simulink model "Latest_Greatest"  (R2022a)
settings: Solver=ode4  StartTime=0  StopTime=15  FixedStep=DeltaT  RelTol=1e-3  EnableMultiTasking=on
InitFcn:
  | % Dynamics Simulation          DA Cole
  | clear all;close all;clc;warning off all;
  | 
  | open('pitchyaw.mat');
  | 
  | % Simulation run parameters
  | %Rate=34.3;  DeltaT=1/Rate;
  | %Rate=40;  DeltaT=1/Rate;
  | %Rate=100;  DeltaT=1/Rate;
  | %Rate=130; DeltaT=1/Rate;
  | %Rate=90; DeltaT=1/Rate;
  | %Rate=110; DeltaT=1/Rate;
  | %Rate=120; DeltaT=1/Rate;
  | %Rate=115; DeltaT=1/Rate;
  | %Rate=125; DeltaT=1/Rate;
  | Rate=117; DeltaT=1/Rate;
  | 
  | 
  | % Maneuver Parameters
  | roll=10;  pitch=-30; yaw=30;   roll=roll*pi/180; pitch=pitch*pi/180; yaw=yaw*pi/180;
  | SlewTime=5;   SACengage=0;
  | 
  | %Constants0
  | Re=6371.2e3;mu=398601.2e9;          %earth radius and universal gravitation constant
  | 
  | %Spacecraft orbit
  | h=0;                                     %orbit altitude
  | R=Re+h;                             %orbit radius from center of earth
  | we=0.000072921158553;   %earth's angular velocity rad/solar sec(Vallado)
  | wo=sqrt(mu/(Re+h)^3);        %orbit angular velocity
  | incln=36.6001*pi/180;          %Inclination assumed Monterey Latitude
  | epsilon=12*pi/180;  alphao=0;
  | uo=0; nuo=0;                        %Start S/C beneath subsolar point
  | beta=60; gamma=1.5;
  | a=0.545491852; b=0.314939867;  c=0.704226952;   %Assumed spacecraft rectangular size
  | Area=[b*c a*c a*b];                 %projected area~m^2 in body x,y,z directions
  | density=4.39e-14;
  | kpre=-9.9639/24/3600/180*pi*0;      %nodal precession constant assumed zero here
  | wn=kpre*(Re/(Re+h))^3.5*cos(incln); %nodal precession (zero eccentricity)
  | V=wo*(Re+h);
  | rho=asin(Re/(h+Re));                %earth angular radius
  | Cd=2.5;     psun=4.5E-6;            %Drag coefficient and solar pressure constant~N/m^2
  | Kaero=-0.5*Cd*V^2;   Psolar=2*psun;  %constants for aero and solar torque calculation
  | dL=[0.002 0.002 0.008];             %predicted distance between cp and cg
  | Kme=2.3390e-005;
  | 
  | %Spacecraft Magnetic Properties (assumed)
  | mresid=[0 0 0.01];                  %Spacecraft residual magnetic moment
  | M=mresid;                           %Magnetic unit dipole vector
  | K=7.943e15;
  | 
  | % ACTUAL Spacecraft Inertia conditions
  | Ix=90;   Iy=100;   Iz=250 ;
  | Ixy=-10;  Iyz=20;  Ixz=-10;
  | Imo=[Ix -Ixy -Ixz;
  |        -Ixy  Iy  -Iyz;
  |        -Ixz -Iyz  Iz];                  %Moment of inertia matrix
  | Iinv=inv(Imo);                      %Moment of inertia inverse goes in dynamics block
  | 
  | %Spacecraft initial Euler state angles and rates
  | ... (+68 lines)
StopFcn:
  | if flag==0; Hcmg=Hcmg;else;Hcmg=HcmgMP;end;
  | Hxcmg=[];Hycmg=[];Hzcmg=[];CondA=[]; CondA_MP=[];t=[]; SingPt=[];DetA=[];
  | for i=1:max(size(A));  t=[t i*DeltaT];  H=Hcmg(:,:,i); Hx=H(1,:);  Hy=H(2,:);  Hz=H(3,:);
  | detA=det(A(:,1:3,i));Hxcmg=[Hxcmg Hx];  Hycmg=[Hycmg Hy];  Hzcmg=[Hzcmg Hz];
  | CONDA=cond(A(:,:,i));
  | DetA=[DetA detA]; DetA=1./DetA;
  | CondA=[CondA CONDA];end;   %CondA=CondA./max(CondA); DetA=DetA./max(DetA);
  | Hmag=sqrt(Hxcmg.^2+Hycmg.^2+Hzcmg.^2);x=(max(t)-DeltaT);
  | 
  | InvCondA;
  | 
  | if flag==0; MaxInvCond=min(1./CondA(10*Rate+1:end));DELTA=delta;DELTAdot=deltadot;
  | else; MaxInvCond=min(1./CondA_MP(10*Rate+1:end));DELTA=delta_MP;DELTAdot=deltadot_MP;Hcmg=HcmgMP;end;
  | 
  | ERROR=(trajectory*180/pi-Euler);
  | 
  | figure(1); wdotTrajectory=[CMDTrajectory(:,1) CMDTrajectory(:,2) CMDTrajectory(:,3)];  wTrajectory=[CMDTrajectory(:,4) CMDTrajectory(:,5) CMDTrajectory(:,6)]; ThetaTrajectory=180/pi.*[trajectory(:,1) trajectory(:,2) trajectory(:,3)];
  | subplot(3,1,1); plot(t,wdotTrajectory,'linewidth',2); axis tight; grid; ylabel('\omega^d^o^t_C_M_D (deg)','fontsize',16); title('Desired Angle, Rate, Acceleration Trajectories','fontsize',16);   set(gca,'XTick',0:2:15);     set(gca,'XTickLabel',{' ',' ',' ',' ',' ',' ',' ',' ','15'});
  | subplot(3,1,2); plot(t,wTrajectory,'linewidth',2); axis tight; grid; ylabel('\omega_C_M_D (deg)','fontsize',16);set(gca,'XTick',0:2:15);     set(gca,'XTickLabel',{' ',' ',' ',' ',' ',' ',' ',' ','15'});
  | subplot(3,1,3); plot(t,ThetaTrajectory,'linewidth',2); axis tight; grid; ylabel('\theta_C_M_D (deg)','fontsize',16); xlabel('time (sec)','fontsize',16);
  | 
  | %figure(2);
  | %subplot(2,1,1);plot(t,Hmag,'LineWidth',3);   ylabel('|H_c_m_g|','Fontsize',16);grid;axis([0,x,0,3]); set(gca,'fontsize',16);set(gca,'XTickLabel',{' ',' ',' ',' ',' ',' ',' ',' ','15'});
  | %subplot(2,1,2);plot(t,InvCondA,'linewidth',3);grid;xlabel('t(sec)','fontsize',14,'fontname','times');ylabel('Cond[A]','fontsize',14,'fontname','times');axis([0,max(t),0,21.82]); set(gca,'fontsize',16);
  | 
  | DELTA1=DELTA(1,:);DELTA2=DELTA(2,:);DELTA3=DELTA(3,:);DELTA4=DELTA(4,:);
  | DELTAdot1=DELTAdot(1,:);DELTAdot2=DELTAdot(2,:);DELTAdot3=DELTAdot(3,:);DELTAdot4=DELTAdot(4,:);
  | 
  | %figure(3);subplot(4,1,1);plot(t,DELTA1,'LineWidth',3); title('Gimbal Angles','fontsize',16);ylabel('\theta_1(deg)','Fontsize',14);grid;axis tight; set(gca,'XTickLabel',{' ',' ',' ',' ',' ',' ',' ',' ','15'});set(gca,'fontsize',16);
  | %subplot(4,1,2);plot(t,DELTA2,'LineWidth',3); ylabel('\theta_2(deg)','Fontsize',16);grid;axis tight; set(gca,'XTickLabel',{' ',' ',' ',' ',' ',' ',' ',' ','15'});set(gca,'fontsize',16);
  | %subplot(4,1,3);plot(t,DELTA3,'LineWidth',3); ylabel('\theta_3(deg)','Fontsize',16);grid;axis tight; set(gca,'XTickLabel',{' ',' ',' ',' ',' ',' ',' ',' ','15'});set(gca,'fontsize',16);
  | %subplot(4,1,4);plot(t,InvCondA,'linewidth',3);grid;xlabel('t(sec)','fontsize',14,'fontname','times');ylabel('Cond[A]','fontsize',14,'fontname','times');axis([0,max(t),0,21.82]); set(gca,'fontsize',16);
  | 
  | %figure(4);subplot(4,1,1);plot(t,DELTAdot1,'LineWidth',3);  title('Gimbal Angle RATES','fontsize',16); ylabel('\theta_d_o_t_1(rad/s)','Fontsize',16);grid; axis([0,x,-pi*1.1,pi*1.1]);   set(gca,'XTickLabel',{' ',' ',' ',' ',' ',' ',' ',' ','15'});set(gca,'fontsize',16);
  | %subplot(4,1,2);plot(t,DELTAdot2,'LineWidth',3);   ylabel('\theta_d_o_t_2(rad/s)','Fontsize',16);grid;axis([0,x,-pi*1.1,pi*1.1]);   set(gca,'XTickLabel',{' ',' ',' ',' ',' ',' ',' ',' ','15'});   set(gca,'fontsize',16);
  | %subplot(4,1,3);plot(t,DELTAdot3,'LineWidth',3);   ylabel('\theta_d_o_t_3(rad/s)','Fontsize',16);grid;axis([0,x,-pi*1.1,pi*1.1]); set(gca,'XTickLabel',{' ',' ',' ',' ',' ',' ',' ',' ','15'});set(gca,'fontsize',16);
  | %subplot(4,1,4);plot(t,InvCondA,'linewidth',3);grid;xlabel('t(sec)','fontsize',14,'fontname','times');ylabel('Cond[A]','fontsize',14,'fontname','times');axis([0,max(t),0,21.82]); set(gca,'fontsize',16);
  | 
  | %figure(5);
  | %subplot(4,1,1);plot(t,Hxcmg,'linewidth',3);axis([0,x,-3.25,3.25]);grid;ylabel('h_x/|h|','fontsize',16);title('Normalized Momentum','fontsize',16);set(gca,'XTickLabel',{' ',' ',' ',' ',' ',' ',' ',' ','15'});set(gca,'fontsize',16);
  | %subplot(4,1,2);plot(t,Hycmg,'linewidth',3);axis([0,x,-3.25,3.25]);grid;ylabel('h_y/|h|','fontsize',16);set(gca,'XTickLabel',{' ',' ',' ',' ',' ',' ',' ',' ','15'});set(gca,'fontsize',16);
  | %subplot(4,1,3);plot(t,Hzcmg,'linewidth',3);axis([0,x,-3.25,3.25]);grid;ylabel('h_z/|h|','fontsize',16);  set(gca,'XTickLabel',{' ',' ',' ',' ',' ',' ',' ',' ','15'});set(gca,'fontsize',16);
  | %subplot(4,1,4);plot(t,InvCondA,'linewidth',3);grid;xlabel('t(sec)','fontsize',14,'fontname','times');ylabel('Cond[A]','fontsize',14,'fontname','times');axis([0,max(t),0,21.82]); set(gca,'fontsize',16);
  | 
  | %figure(6); EulerX=Euler(:,1);EulerY=Euler(:,2);EulerZ=Euler(:,3);
  | %subplot(4,1,1);plot(t,EulerX,'linewidth',3); axis([0,x,min(EulerX)*5,max(EulerX)*5]);grid;ylabel('\phi(deg)','fontsize',16);title('True Euler Angles','fontsize',14);  set(gca,'XTickLabel',{' ',' ',' ',' ',' ',' ',' ',' ','15'});  set(gca,'fontsize',16);
  | %subplot(4,1,2);plot(t,EulerY,'linewidth',3);  axis([0,x,min(EulerY)*5,max(EulerY)*5]); grid;ylabel('\theta(deg)','fontsize',14);  set(gca,'XTickLabel',{' ',' ',' ',' ',' ',' ',' ',' ','15'}); set(gca,'fontsize',16);
  | %subplot(4,1,3);plot(t,EulerZ,'linewidth',3);axis([0,x,min(EulerZ)*1.25,max(EulerZ)*1.25]);grid;  ylabel('\psi(deg)','fontsize',14);  set(gca,'XTickLabel',{' ',' ',' ',' ',' ',' ',' ',' ','15'});  set(gca,'fontsize',16);
  | %subplot(4,1,4);plot(t,InvCondA,'linewidth',3);grid;xlabel('t(sec)','fontsize',14,'fontname','times');ylabel('Cond[A]','fontsize',14,'fontname','times');axis([0,max(t),0,21.82]); set(gca,'fontsize',16);
  | 
  | EX=ERROR(:,1);  EY=ERROR(:,2);     EZ=ERROR(:,3);
  | MeanXerror=mean(EX); Xmean=num2str(MeanXerror); xmean=['\mu_\phi=', Xmean];
  | STDx=std(EX);Xsigma=num2str(STDx);SigmaX=['    \sigma_x=' Xsigma];  xlegend=[xmean, SigmaX];
  | MeanYerror=mean(EY); Ymean=num2str(MeanYerror); ymean=['\mu_\theta=', Ymean];
  | STDy=std(EY); Ysigma=num2str(STDy);SigmaY=['    \sigma_y=' Ysigma]; ylegend=[ymean, SigmaY];
  | MeanZerror=mean(EZ); Zmean=num2str(MeanZerror); zmean=['\mu_\psi=', Zmean];
  | STDz=std(EZ);Zsigma=num2str(STDz);SigmaZ=['    \sigma_z=' Zsigma]; zlegend=[zmean, SigmaZ];
  | MeanError=[MeanXerror MeanYerror MeanZerror];  StdDev=[STDx STDy STDz];
  | 
  | figure(7);
  | ... (+83 lines)
undefined symbols (not defined in the file): magnitude, svd
libraries: aerospace x6, vrlib x4, simulink_need_slupdate x2, dspadpt3 x2, dspinverses x1
(part 2 of 2)

== system Latest_Greatest/Subsystem5/OBSERVERS (MASK THIS SUBSYSTEM AS CLASS DEMO)1 ==
  Full State Feedback : Inport
  Demux : Demux  Outputs=2
  Subsystem : Subsystem
      mask Display: disp('Luenberger & PID Observers')
  Terminator : Terminator
  Estimated full state feedback (Euler-rad) : Outport  VectorParamsAs1DForOutWhenUnconnected=off
  wires:
  Demux/1 -> Subsystem/1(Euler Angle (rad))
  Demux/2 -> Terminator/1
  Subsystem/1(Estimated Full State Feedback) -> Estimated full state feedback (Euler-rad)/1
  Full State Feedback/1 -> Demux/1

== system Latest_Greatest/Subsystem5/Subsystem2 ==
  note: Noisy Sensor
  Full State Feedback : Inport
  Random Number : RandomNumber  Variance=NoiseVariance  SampleTime=0
  Sum1 : Sum  Inputs=|++
  Noisy State Feedback : Outport  VectorParamsAs1DForOutWhenUnconnected=off
  wires:
  Random Number/1 -> Sum1/2
  Sum1/1 -> Noisy State Feedback/1
  Full State Feedback/1 -> Sum1/1

== system Latest_Greatest/Subsystem5/Subsystem4 ==
  Full State Feedback : Inport
  Demux : Demux  Outputs=2
  Filter Error (deg) : Scope
      settings: StopFcn=|
      | %Simulink figure properties
      | shh=get(0,'ShowHiddenHandles');
      | set(0,'ShowHiddenHandles','On')
      | set(gcf,'menubar','figure')
      | set(gcf,'CloseRequestFcn','closereq')
      | set(gcf,'DefaultLineClipping','Off')
      | set(0,'ShowHiddenHandles',shh)
  Filtered Euler Angles (deg) : Scope
      settings: StopFcn=|
      | %Simulink figure properties
      | shh=get(0,'ShowHiddenHandles');
      | set(0,'ShowHiddenHandles','On')
      | set(gcf,'menubar','figure')
      | set(gcf,'CloseRequestFcn','closereq')
      | set(gcf,'DefaultLineClipping','Off')
      | set(0,'ShowHiddenHandles',shh)
  Kalman Filter : dspadpt3/Kalman Filter  num_targets=1  sourceEnable=Always  isReset=on  X=zeros([3, 1])  P=10*eye(3)  A=eye(3)  sourceMeasure=Specify via Dialog  H=eye(3)  Q=0.05*eye(3)  R=eye(3)  isOutputEstMeasure=off  isOutputEstState=on  isOutputEstError=off  isOutputPrdMeasure=off  isOutputPrdState=off  isOutputPrdError=off
      settings: SourceProductBaseCode=DS
  Kalman Filter1 : dspadpt3/Kalman Filter  num_targets=1  sourceEnable=Always  isReset=on  X=zeros([3, 1])  P=10*eye(3)  A=eye(3)  sourceMeasure=Specify via Dialog  H=eye(3)  Q=0.05*eye(3)  R=eye(3)  isOutputEstMeasure=off  isOutputEstState=on  isOutputEstError=off  isOutputPrdMeasure=off  isOutputPrdState=off  isOutputPrdError=off
      settings: SourceProductBaseCode=DS
  Mux : Mux  Inputs=2
  Reshape : Reshape
  Sum3 : Sum  Inputs=|+-
  To Workspace : ToWorkspace  VariableName=FilteredEuler  SampleTime=-1
  To Workspace2 : ToWorkspace  VariableName=KalmanEstimationError  SampleTime=-1
  degrees-to-radians2 : Gain  Gain=180/pi
  Out1 : Outport  VectorParamsAs1DForOutWhenUnconnected=off
  wires:
  [ActualEuler] -> Sum3/1
  Reshape/1 -> Sum3/2
  Sum3/1 -> Filter Error (deg)/1, To Workspace2/1
  degrees-to-radians2/1 -> Reshape/1, Filtered Euler Angles (deg)/1, To Workspace/1
  Kalman Filter/1 -> degrees-to-radians2/1, Mux/1
  Demux/2 -> Kalman Filter1/1
  Full State Feedback/1 -> Demux/1
  Demux/1 -> Kalman Filter/1
  Mux/1 -> Out1/1
  Kalman Filter1/1 -> Mux/2

== system Latest_Greatest/Subsystem5/Subsystem5 ==
  note: See Bong Wie
      | Generalized Second Order Filters
      | 2nd Edition pg 137
  u : Inport
  Demux : Demux  Outputs=6
  Mux : Mux  Inputs=6
  Transfer Fcn{,1..5} (6 alike) : TransferFcn  Numerator="[1/wz^2   2*dampZ/wz  1]"  Denominator="[1/wp^2   2*dampP/wp  1]"
  u(filtered) : Outport  VectorParamsAs1DForOutWhenUnconnected=off
  wires:
  Mux/1 -> u(filtered)/1
  u/1 -> Demux/1
  Transfer Fcn/1 -> Mux/1
  Transfer Fcn1/1 -> Mux/2
  Transfer Fcn2/1 -> Mux/3
  Transfer Fcn3/1 -> Mux/4
  Transfer Fcn4/1 -> Mux/5
  Transfer Fcn5/1 -> Mux/6
  Demux/1 -> Transfer Fcn/1
  Demux/2 -> Transfer Fcn1/1
  Demux/3 -> Transfer Fcn2/1
  Demux/4 -> Transfer Fcn3/1
  Demux/5 -> Transfer Fcn4/1
  Demux/6 -> Transfer Fcn5/1

== system Latest_Greatest/CMGs/CMG Steering Logic1/Subsystem ==
  "[A]" : Inport
  Divide : Product  Inputs=/*
  max (SVD[A]) : MATLABFcn  MATLABFcn=max(svd(u))
  min (SVD[A]) : MATLABFcn  MATLABFcn=min(svd(u))
  1/Cond[A] : Outport  VectorParamsAs1DForOutWhenUnconnected=off
  wires:
  Divide/1 -> 1/Cond[A]/1
  max (SVD[A])/1 -> Divide/2
  min (SVD[A])/1 -> Divide/1
  "[A]"/1 -> max (SVD[A])/1, min (SVD[A])/1

== system Latest_Greatest/CMGs/CMG Steering Logic1/Subsystem1 ==
  delta : Inport
  3x4 : Reshape  OutputDimensionality=Customize  OutputDimensions=[3,4]
  "[A] Matrix" : MATLABFcn  MATLABFcn="[ -cos(beta(1))*cos(u(1)),  sin(u(2)), cos(beta(3))*cos(u(3)), 0   ;  -sin(u(1)),  -cos(beta(2))*cos(u(2)),  sin(u(3)),   0;  sin(beta(1))*cos(u(1)),  sin(beta(2))*cos(u(2)),  sin(beta(3))*cos(u(3)),   0  ]"
  "[A]" : Outport  VectorParamsAs1DForOutWhenUnconnected=off
  wires:
  "[A] Matrix"/1 -> 3x4/1
  delta/1 -> "[A] Matrix"/1
  3x4/1 -> "[A]"/1

== system Latest_Greatest/CMGs/CMG Steering Logic1/Subsystem3 ==
  1/Cond[A] : Inport
  deltaDot : Inport  Port=2
  Switch : Switch  Threshold=2.21  SaturateOnIntegerOverflow=off  InputSameDT=off
  Unit Delay : UnitDelay  SampleTime=-1  HasFrameUpgradeWarning=on
  Out1 : Outport  VectorParamsAs1DForOutWhenUnconnected=off
  wires:
  1/Cond[A]/1 -> Switch/2
  deltaDot/1 -> Switch/1
  Switch/1 -> Unit Delay/1, Out1/1
  Unit Delay/1 -> Switch/3

== system Latest_Greatest/CMGs/Subsystem1/Displays ==
  Tc : Inport
  d : Inport  Port=2
  u : Inport  Port=3
  -3 : Gain  Gain=-1  SaturateOnIntegerOverflow=on  OutDataTypeStr=Inherit: Same as input  ParamDataTypeStr=Inherit: Same as input
  Demux : Demux
  Demux1 : Demux  Outputs=3
  Demux2 : Demux  Outputs=3
  Sum : Sum  Inputs=+-|
  Tcmg : Scope  NumInputPorts=3
  To Workspace : ToWorkspace  VariableName=ControlError  SampleTime=-1
  d. : Scope  NumInputPorts=4
  uc : Scope  NumInputPorts=3
  wires:
  d/1 -> Demux/1
  u/1 -> -3/1
  Demux/4 -> d./4
  Demux/3 -> d./3
  Demux/2 -> d./2
  Demux/1 -> d./1
  -3/1 -> Demux1/1, Sum/1
  Tc/1 -> Demux2/1, Sum/2
  Demux2/1 -> Tcmg/1
  Demux2/2 -> Tcmg/2
  Demux2/3 -> Tcmg/3
  Demux1/1 -> uc/1
  Demux1/2 -> uc/2
  Demux1/3 -> uc/3
  Sum/1 -> To Workspace/1

== system Latest_Greatest/CMGs/Subsystem1/Subsystem ==
  SAC/MP : Inport
  Demux : Demux  Outputs=8
  Mux : Mux  Inputs=3
  Mux1 : Mux
  To Workspace : ToWorkspace  VariableName=flag  SampleTime=-1
  Torque : Outport  VectorParamsAs1DForOutWhenUnconnected=off
  GimbalAngles : Outport  Port=2  VectorParamsAs1DForOutWhenUnconnected=off
  wires:
  SAC/MP/1 -> Demux/1
  Demux/8 -> To Workspace/1
  Demux/1 -> Mux/1
  Demux/2 -> Mux/2
  Demux/3 -> Mux/3
  Demux/4 -> Mux1/1
  Demux/5 -> Mux1/2
  Demux/6 -> Mux1/3
  Demux/7 -> Mux1/4
  Mux1/1 -> GimbalAngles/1
  Mux/1 -> Torque/1

== system Latest_Greatest/CMGs/Subsystem1/Subsystem2 ==
  note: Gimbal Angles
  note: u
  note: flag
  u : Inport
  gimbal angles : Inport  Port=2
  Constant1 : Constant
  Mux1 : Mux  Inputs=3
  MP : Outport  VectorParamsAs1DForOutWhenUnconnected=off
  wires:
  u/1 -> Mux1/1
  Constant1/1 -> Mux1/3
  Mux1/1 -> MP/1
  gimbal angles/1 -> Mux1/2

== system Latest_Greatest/CMGs/Subsystem3/Subsystem1 ==
  note: e(s)
  note: w
  note: (s)
  note: q
  note: (s)
  note: u(s)
  note: *
  note: q
  note: (s)
  note: w
  note: *
  note: (s)
  Full State Feedback : Inport
  FullCMDTraj : Inport  Port=2
  Demux : Demux  Outputs=2
  Demux1 : Demux  Outputs=2
  Integrator9 : Integrator
  Subsystem25 : Subsystem
      mask Display: disp('Ki')
  Subsystem26 : Subsystem
      mask Display: disp('Kp')
  Subsystem27 : Subsystem
      mask Display: disp('Kd')
  Sum12 : Sum  Inputs=|+-
  Sum14 : Sum  Inputs=+++
  Sum15 : Sum  Inputs=|+-
  "Control, u-fb" : Outport  VectorParamsAs1DForOutWhenUnconnected=off
  wires:
  Sum14/1 -> "Control, u-fb"/1
  Demux/1 -> Sum12/2
  Sum15/1 -> Subsystem27/1(In1)
  Integrator9/1 -> Subsystem25/1(In1)
  Sum12/1 -> Subsystem26/1(In1), Integrator9/1
  Subsystem27/1(Out1) -> Sum14/3
  Subsystem26/1(Out1) -> Sum14/2
  Subsystem25/1(Out1) -> Sum14/1
  Demux1/2 -> Sum15/1
  Demux1/1 -> Sum12/1
  Full State Feedback/1 -> Demux/1
  Demux/2 -> Sum15/2
  FullCMDTraj/1 -> Demux1/1

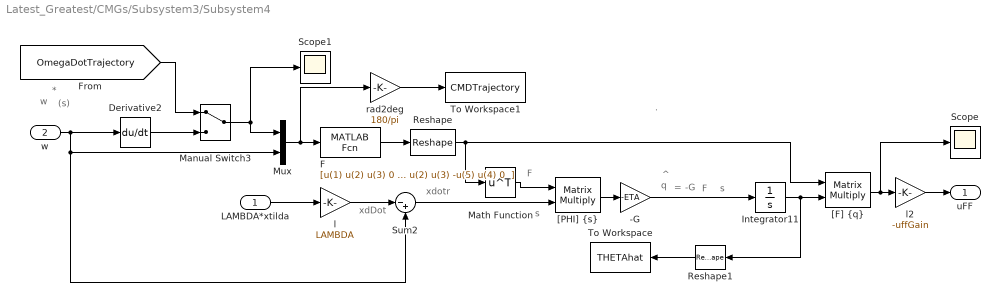
== system Latest_Greatest/CMGs/Subsystem3/Subsystem4 ==
  note: xdotr
  note: s
  note: xdDot
  note: F
  note: -G
  note: F
  note: s
  note: =
  note: .
  note: ^
  note: q
  note: *
  note: (s)
  note: w
  LAMBDA*xtilda : Inport
  w : Inport  Port=2
  -G : Gain  Gain=-ETA  SaturateOnIntegerOverflow=on  OutDataTypeStr=Inherit: Same as input  ParamDataTypeStr=Inherit: Same as input
  Derivative2 : Derivative
  F : MATLABFcn  MATLABFcn="[u(1) u(2) u(3) 0 0 0 0 -u(6) u(5);  0 u(1) 0 u(2) u(3) 0 u(6) 0 u(4);  0 0 u(1) 0 u(2) u(3) -u(5) u(4) 0  ]"
  Integrator11 : Integrator  InitialCondition=THETAo
  Manual Switch3 : ManualSwitch
  Math Function : Math  Operator=transpose  SignedPower=on
  Mux : Mux  Inputs=2
  Reshape : Reshape  OutputDimensionality=Customize  OutputDimensions=[3,9]
  Reshape1 : Reshape  OutputDimensions=[1,9]
  Scope : Scope
  Scope1 : Scope
  Sum2 : Sum  Inputs=|-+  SaturateOnIntegerOverflow=on
  To Workspace : ToWorkspace  VariableName=THETAhat  SampleTime=-1
  To Workspace1 : ToWorkspace  VariableName=CMDTrajectory  SampleTime=-1
  "[F] {q}" : Product  Multiplication=Matrix(*)  SaturateOnIntegerOverflow=on  OutDataTypeStr=Inherit: Same as first input
  "[PHI] {s}" : Product  Multiplication=Matrix(*)  SaturateOnIntegerOverflow=on  OutDataTypeStr=Inherit: Same as first input
  l : Gain  Gain=LAMBDA  SaturateOnIntegerOverflow=on  OutDataTypeStr=Inherit: Same as input  ParamDataTypeStr=Inherit: Same as input
  l2 : Gain  Gain=-uffGain  SaturateOnIntegerOverflow=on  OutDataTypeStr=Inherit: Same as input  ParamDataTypeStr=Inherit: Same as input
  rad2deg : Gain  Gain=180/pi  SaturateOnIntegerOverflow=on  OutDataTypeStr=Inherit: Same as input  ParamDataTypeStr=Inherit: Same as input
  uFF : Outport  VectorParamsAs1DForOutWhenUnconnected=off
  wires:
  LAMBDA*xtilda/1 -> l/1
  l/1 -> Sum2/1
  Sum2/1 -> "[PHI] {s}"/2
  "[PHI] {s}"/1 -> -G/1
  F/1 -> Reshape/1
  w/1 -> Derivative2/1, Mux/2, Sum2/2
  Mux/1 -> F/1, rad2deg/1
  -G/1 -> Integrator11/1
  "[F] {q}"/1 -> l2/1, Scope/1
  Reshape/1 -> "[F] {q}"/1, Math Function/1
  Math Function/1 -> "[PHI] {s}"/1
  Reshape1/1 -> To Workspace/1
  Integrator11/1 -> "[F] {q}"/2, Reshape1/1
  rad2deg/1 -> To Workspace1/1
  l2/1 -> uFF/1
  Manual Switch3/1 -> Mux/1, Scope1/1
  [OmegaDotTrajectory] -> Manual Switch3/1
  Derivative2/1 -> Manual Switch3/2

== system Latest_Greatest/Subsystem2/Subsystem/Gravity Gradient ==
  note: Gravity Gradient Disturbances
  DCM : Inport
  3*mu/Ro^3 : Gain  Gain=3*mu/(h+Re)^3  Multiplication=Matrix(K*u)  SaturateOnIntegerOverflow=on  OutDataTypeStr=Inherit: Same as input  ParamDataTypeStr=Inherit: Same as input
  3x3 cross product : aerospace/Axes Transformations/3x3 cross product
      settings: SourceProductBaseCode=SL
  Body Inertia : Gain  Gain=Imo  Multiplication=Matrix(K*u)  SaturateOnIntegerOverflow=on  OutDataTypeStr=Inherit: Same as input  ParamDataTypeStr=Inherit: Same as input
  Select ci3 : Subsystem
  Tgg : Outport
  wires:
  Body Inertia/1 -> 3x3 cross product/2
  3*mu/Ro^3/1 -> Tgg/1
  3x3 cross product/1 -> 3*mu/Ro^3/1
  Select ci3/1(U(E)) -> 3x3 cross product/1, Body Inertia/1
  DCM/1 -> Select ci3/1(U)

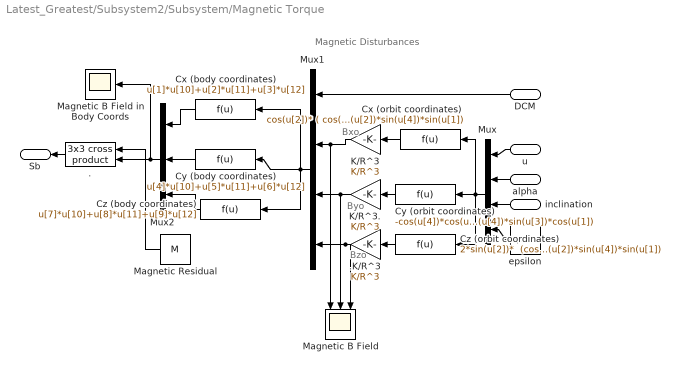
== system Latest_Greatest/Subsystem2/Subsystem/Magnetic Torque ==
  note: Magnetic Disturbances
  note: Bzo
  note: Byo
  note: Bxo
  DCM : Inport
  alpha : Inport  Port=2
  inclination : Inport  Port=3
  u : Inport  Port=4
  . : aerospace/Axes Transformations/3x3 cross product
      settings: SourceProductBaseCode=SL
  .K/R^3 : Gain  Gain=K/R^3  SaturateOnIntegerOverflow=on  OutDataTypeStr=Inherit: Same as input  ParamDataTypeStr=Inherit: Same as input
  Cx (orbit coordinates) : Fcn  Expr="cos(u[2])* ( cos(u[4])*sin(u[3])-sin(u[4])*cos(u[3])*cos(u[1])  ) - sin(u[2])*sin(u[4])*sin(u[1])"
  Cx (body coordinates) : Fcn  Expr=u[1]*u[10]+u[2]*u[11]+u[3]*u[12]
  Cy (orbit coordinates) : Fcn  Expr=-cos(u[4])*cos(u[3])-sin(u[4])*sin(u[3])*cos(u[1])
  Cy (body coordinates) : Fcn  Expr=u[4]*u[10]+u[5]*u[11]+u[6]*u[12]
  Cz (orbit coordinates) : Fcn  Expr="2*sin(u[2])*  (cos(u[4])*sin(u[3])-sin(u[4])*cos(u[3])*cos(u[1]) ) + 2*cos(u[2])*sin(u[4])*sin(u[1])"
  Cz (body coordinates) : Fcn  Expr=u[7]*u[10]+u[8]*u[11]+u[9]*u[12]
  K/R^3 : Gain  Gain=K/R^3  SaturateOnIntegerOverflow=on  OutDataTypeStr=Inherit: Same as input  ParamDataTypeStr=Inherit: Same as input
  K/R^3. : Gain  Gain=K/R^3  SaturateOnIntegerOverflow=on  OutDataTypeStr=Inherit: Same as input  ParamDataTypeStr=Inherit: Same as input
  Magnetic B Field : Scope  NumInputPorts=3
  Magnetic B Field in Body Coords : Scope
  Magnetic Residual : Constant  Value=M
  Mux : Mux
  Mux1 : Mux
  Mux2 : Mux  Inputs=3
  epsilon : Constant  Value=epsilon
  Sb : Outport
  wires:
  Mux2/1 -> Magnetic B Field in Body Coords/1, ./2
  Magnetic Residual/1 -> ./1
  ./1 -> Sb/1
  Cz (body coordinates)/1 -> Mux2/3
  Cx (body coordinates)/1 -> Mux2/1
  Cy (body coordinates)/1 -> Mux2/2
  Mux1/1 -> Cz (body coordinates)/1, Cx (body coordinates)/1, Cy (body coordinates)/1
  .K/R^3/1 -> Mux1/4, Magnetic B Field/3
  K/R^3./1 -> Magnetic B Field/2, Mux1/3
  K/R^3/1 -> Magnetic B Field/1, Mux1/2
  DCM/1 -> Mux1/1
  Cz (orbit coordinates)/1 -> .K/R^3/1
  Cy (orbit coordinates)/1 -> K/R^3./1
  Cx (orbit coordinates)/1 -> K/R^3/1
  epsilon/1 -> Mux/4
  Mux/1 -> Cz (orbit coordinates)/1, Cx (orbit coordinates)/1, Cy (orbit coordinates)/1
  inclination/1 -> Mux/3
  alpha/1 -> Mux/2
  u/1 -> Mux/1

== system Latest_Greatest/Subsystem2/Subsystem/Orbit parameters ==
  note: Orbit parameters
  note: nu=nuo-alpha
  note: alpha
  Clock : Clock
  Sum2 : Sum  Inputs=-+  InputSameDT=on  SaturateOnIntegerOverflow=on  OutDataTypeStr=Inherit: Same as first input
  Sum3 : Sum  InputSameDT=on  SaturateOnIntegerOverflow=on  OutDataTypeStr=Inherit: Same as first input
  Sum4 : Sum  InputSameDT=on  SaturateOnIntegerOverflow=on  OutDataTypeStr=Inherit: Same as first input
  alphao : Constant  Value=alphao
  inclination : Constant  Value=incln
  nuo : Constant  Value=nuo
  udot*t=t/365/360 : Gain  Gain=1/365.242/360  SaturateOnIntegerOverflow=on  OutDataTypeStr=Inherit: Same as input  ParamDataTypeStr=Inherit: Same as input
  uo : Constant  Value=uo
  wo : Gain  Gain=wo  SaturateOnIntegerOverflow=on  OutDataTypeStr=Inherit: Same as input  ParamDataTypeStr=Inherit: Same as input
  alpha : Outport
  incln : Outport  Port=2
  u : Outport  Port=3
  nu : Outport  Port=4
  wires:
  Sum3/1 -> u/1
  inclination/1 -> incln/1
  Sum2/1 -> nu/1
  Sum4/1 -> alpha/1, Sum2/2
  nuo/1 -> Sum2/1
  uo/1 -> Sum3/2
  udot*t=t/365/360/1 -> Sum3/1
  wo/1 -> Sum4/2
  alphao/1 -> Sum4/1
  Clock/1 -> udot*t=t/365/360/1, wo/1

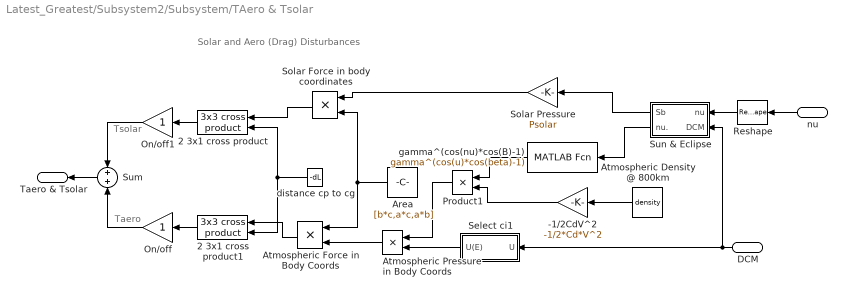
== system Latest_Greatest/Subsystem2/Subsystem/TAero & Tsolar ==
  note: Solar and Aero (Drag) Disturbances
  note: Tsolar
  note: Taero
  nu : Inport
  DCM : Inport  Port=2
  -1/2CdV^2 : Gain  Gain=-1/2*Cd*V^2  SaturateOnIntegerOverflow=on  OutDataTypeStr=Inherit: Same as input  ParamDataTypeStr=Inherit: Same as input
  2 3x1 cross product : aerospace/Axes Transformations/3x3 cross product
      settings: SourceProductBaseCode=SL
  2 3x1 cross product1 : aerospace/Axes Transformations/3x3 cross product
      settings: SourceProductBaseCode=SL
  Area : Constant  Value=[b*c,a*c,a*b]
  Atmospheric Density @ 800km : Constant  Value=density
  Atmospheric Force in Body Coords : Product  SaturateOnIntegerOverflow=on  OutDataTypeStr=Inherit: Same as first input
  Atmospheric Pressure in Body Coords : Product  SaturateOnIntegerOverflow=on  OutDataTypeStr=Inherit: Same as first input
  On/off : Gain  SaturateOnIntegerOverflow=on  OutDataTypeStr=Inherit: Same as input  ParamDataTypeStr=Inherit: Same as input
  On/off1 : Gain  SaturateOnIntegerOverflow=on  OutDataTypeStr=Inherit: Same as input  ParamDataTypeStr=Inherit: Same as input
  Product1 : Product  SaturateOnIntegerOverflow=on  OutDataTypeStr=Inherit: Same as first input
  Reshape : Reshape  OutputDimensionality=Customize  OutputDimensions=[3,1]
  Select ci1 : Subsystem
  Solar Force in body coordinates : Product  SaturateOnIntegerOverflow=on  OutDataTypeStr=Inherit: Same as first input
  Solar Pressure : Gain  Gain=Psolar  SaturateOnIntegerOverflow=on  OutDataTypeStr=Inherit: Same as input  ParamDataTypeStr=Inherit: Same as input
  Sum : Sum  SaturateOnIntegerOverflow=on
  Sun & Eclipse : Subsystem
  distance cp to cg : Constant  Value=-dL
  gamma^(cos(nu)*cos(B)-1) : MATLABFcn  MATLABFcn=gamma^(cos(u)*cos(beta)-1)
  Taero & Tsolar : Outport
  wires:
  Atmospheric Force in Body Coords/1 -> 2 3x1 cross product1/1
  nu/1 -> Reshape/1
  On/off1/1 -> Sum/1
  2 3x1 cross product/1 -> On/off1/1
  2 3x1 cross product1/1 -> On/off/1
  On/off/1 -> Sum/2
  DCM/1 -> Sun & Eclipse/2(DCM), Select ci1/1(U)
  Sun & Eclipse/2(nu.) -> gamma^(cos(nu)*cos(B)-1)/1
  Sun & Eclipse/1(Sb) -> Solar Pressure/1
  Sum/1 -> Taero & Tsolar/1
  distance cp to cg/1 -> 2 3x1 cross product1/2, 2 3x1 cross product/2
  Solar Force in body coordinates/1 -> 2 3x1 cross product/1
  Atmospheric Pressure in Body Coords/1 -> Atmospheric Force in Body Coords/2
  Select ci1/1(U(E)) -> Atmospheric Pressure in Body Coords/2
  Product1/1 -> Atmospheric Pressure in Body Coords/1
  Area/1 -> Atmospheric Force in Body Coords/1, Solar Force in body coordinates/2
  Solar Pressure/1 -> Solar Force in body coordinates/1
  -1/2CdV^2/1 -> Product1/2
  Atmospheric Density @ 800km/1 -> -1/2CdV^2/1
  Reshape/1 -> Sun & Eclipse/1(nu)
  gamma^(cos(nu)*cos(B)-1)/1 -> Product1/1

== system Latest_Greatest/Subsystem3/Subsystem1/121 ==
  note: y
  note: q
  note: f
  DCM : Inport
  Constant : Constant  Value=0
  Mux : Mux  Inputs=3
  atan2(21/12) : Fcn  Expr=atan2(u[4],u[2])
  atan2(21/31) : Fcn  Expr=atan2(u[4],u[7])
  Euler Angles : Outport  VectorParamsAs1DForOutWhenUnconnected=off
  wires:
  Constant/1 -> Mux/3
  atan2(21/31)/1 -> Mux/1
  atan2(21/12)/1 -> Mux/2
  DCM/1 -> atan2(21/31)/1, atan2(21/12)/1
  Mux/1 -> Euler Angles/1

== system Latest_Greatest/Subsystem3/Subsystem1/123 ==
  note: y
  note: q
  note: f
  DCM : Inport
  (31*sin) : Fcn  Expr=u[1]*sin(u[2])
  31 : Fcn  Expr=u[7]
  32 : Fcn  Expr=-u[8]
  Mux : Mux  Inputs=3
  Mux1 : Mux  Inputs=2
  Mux2 : Mux  Inputs=2
  atan2(21/11) : Fcn  Expr=atan2(-u[4],u[1])
  atan2(31/32*sin) : Fcn  Expr=atan2(u[1],u[2])
  atan2(32/33) : Fcn  Expr=atan2(-u[8],u[9])
  Euler Angles : Outport  VectorParamsAs1DForOutWhenUnconnected=off
  wires:
  atan2(21/11)/1 -> Mux/3
  atan2(32/33)/1 -> Mux1/2, Mux/2
  atan2(31/32*sin)/1 -> Mux/1
  DCM/1 -> atan2(21/11)/1, 32/1, 31/1, atan2(32/33)/1
  Mux/1 -> Euler Angles/1
  Mux1/1 -> (31*sin)/1
  31/1 -> Mux1/1
  Mux2/1 -> atan2(31/32*sin)/1
  (31*sin)/1 -> Mux2/1
  32/1 -> Mux2/2

== system Latest_Greatest/Subsystem3/Subsystem1/131 ==
  note: y
  note: q
  note: f
  DCM : Inport
  (11*cos) : Fcn  Expr=u[2]*cos(u[1])
  11 : Fcn  Expr=u[1]
  21 : Fcn  Expr=-u[4]
  Constant : Constant  Value=0
  Mux : Mux  Inputs=3
  Mux1 : Mux  Inputs=2
  Mux2 : Mux  Inputs=2
  atan2((12/11)/cos) : Fcn  Expr=atan2(u[1],u[2])
  atan2(31/21) : Fcn  Expr=atan2(u[7],-u[4])
  Euler Angles : Outport  VectorParamsAs1DForOutWhenUnconnected=off
  wires:
  atan2(31/21)/1 -> Mux2/1, Mux/2
  DCM/1 -> 11/1, 21/1, atan2(31/21)/1
  Mux/1 -> Euler Angles/1
  Constant/1 -> Mux/1
  atan2((12/11)/cos)/1 -> Mux/3
  Mux1/1 -> atan2((12/11)/cos)/1
  (11*cos)/1 -> Mux1/2
  Mux2/1 -> (11*cos)/1
  11/1 -> Mux2/2
  21/1 -> Mux1/1

== system Latest_Greatest/Subsystem3/Subsystem1/132 ==
  note: y
  note: f
  note: q
  note: f
  DCM : Inport
  (21*sin) : Fcn  Expr=u[2]*sin(u[1])
  11 : Fcn  Expr=u[1]
  21 : Fcn  Expr=-u[4]
  Mux : Mux  Inputs=3
  Mux1 : Mux  Inputs=2
  Mux2 : Mux  Inputs=2
  atan2(21/11*sin) : Fcn  Expr=atan2(u[1],u[2])
  atan2(23/22) : Fcn  Expr=atan2(u[6],u[5])
  atan2(31/11) : Fcn  Expr=atan2(u[7],u[1])
  Euler Angles : Outport  VectorParamsAs1DForOutWhenUnconnected=off
  wires:
  atan2(23/22)/1 -> Mux2/1, Mux/2
  DCM/1 -> 11/1, 21/1, atan2(31/11)/1, atan2(23/22)/1
  Mux/1 -> Euler Angles/1
  atan2(31/11)/1 -> Mux/1
  atan2(21/11*sin)/1 -> Mux/3
  Mux1/1 -> atan2(21/11*sin)/1
  Mux2/1 -> (21*sin)/1
  (21*sin)/1 -> Mux1/1
  21/1 -> Mux2/2
  11/1 -> Mux1/2

== system Latest_Greatest/Subsystem3/Subsystem1/212 ==
  note: y
  note: f
  note: q
  note: f
  DCM : Inport
  (22*cos) : Fcn  Expr=u[2]*cos(u[1])
  22 : Fcn  Expr=u[5]
  32 : Fcn  Expr=-u[8]
  Constant : Constant  Value=0
  Mux : Mux  Inputs=3
  Mux1 : Mux  Inputs=2
  Mux2 : Mux  Inputs=2
  atan2(12/23) : Fcn  Expr=atan2(u[2],u[6])
  atan2(32/22*cos) : Fcn  Expr=atan2(u[1],u[2])
  Euler Angles : Outport  VectorParamsAs1DForOutWhenUnconnected=off
  wires:
  Constant/1 -> Mux/3
  DCM/1 -> 22/1, atan2(12/23)/1, 32/1
  Mux/1 -> Euler Angles/1
  atan2(12/23)/1 -> Mux2/1, Mux/1
  atan2(32/22*cos)/1 -> Mux/2
  Mux1/1 -> atan2(32/22*cos)/1
  Mux2/1 -> (22*cos)/1
  22/1 -> Mux2/2
  32/1 -> Mux1/1
  (22*cos)/1 -> Mux1/2

== system Latest_Greatest/Subsystem3/Subsystem1/213 ==
  note: y
  note: q
  note: f
  DCM : Inport
  (32*cos) : Fcn  Expr=u[1]*cos(u[2])
  22 : Fcn  Expr=u[5]
  32 : Fcn  Expr=-u[8]
  Mux : Mux  Inputs=3
  Mux1 : Mux  Inputs=2
  Mux2 : Mux  Inputs=2
  atan2(12/22) : Fcn  Expr=atan2(u[2],u[5])
  atan2(31/33) : Fcn  Expr=atan2(u[7],u[9])
  atan2(32/22*cos) : Fcn  Expr=atan2(u[2],u[1])
  Euler Angles : Outport  VectorParamsAs1DForOutWhenUnconnected=off
  wires:
  atan2(12/22)/1 -> Mux1/2, Mux/3
  DCM/1 -> 22/1, atan2(12/22)/1, atan2(31/33)/1, 32/1
  Mux/1 -> Euler Angles/1
  atan2(31/33)/1 -> Mux/1
  atan2(32/22*cos)/1 -> Mux/2
  Mux1/1 -> (32*cos)/1
  32/1 -> Mux1/1
  Mux2/1 -> atan2(32/22*cos)/1
  (32*cos)/1 -> Mux2/2
  22/1 -> Mux2/1

== system Latest_Greatest/Subsystem3/Subsystem1/231 ==
  note: y
  note: f
  note: q
  note: f
  DCM : Inport
  (12*cos) : Fcn  Expr=u[2]*cos(u[1])
  11 : Fcn  Expr=u[1]
  12 : Fcn  Expr=u[2]
  Mux : Mux  Inputs=3
  Mux1 : Mux  Inputs=2
  Mux2 : Mux  Inputs=2
  atan2(12/11*cos) : Fcn  Expr=atan2(u[1],u[2])
  atan2(13/11) : Fcn  Expr=atan2(-u[3],u[1])
  atan2(32/22) : Fcn  Expr=atan2(-u[8],u[5])
  Euler Angles : Outport  VectorParamsAs1DForOutWhenUnconnected=off
  wires:
  atan2(32/22)/1 -> Mux/2
  DCM/1 -> 11/1, 12/1, atan2(13/11)/1, atan2(32/22)/1
  Mux/1 -> Euler Angles/1
  atan2(13/11)/1 -> Mux1/1, Mux/1
  atan2(12/11*cos)/1 -> Mux/3
  Mux1/1 -> (12*cos)/1
  12/1 -> Mux1/2
  (12*cos)/1 -> Mux2/1
  11/1 -> Mux2/2
  Mux2/1 -> atan2(12/11*cos)/1

== system Latest_Greatest/Subsystem3/Subsystem1/232 ==
  note: y
  note: f
  note: q
  note: f
  DCM : Inport
  (22*cos) : Fcn  Expr=u[2]*cos(u[1])
  21 : Fcn  Expr=-u[4]
  22 : Fcn  Expr=u[5]
  Constant : Constant  Value=0
  Mux : Mux  Inputs=3
  Mux1 : Mux  Inputs=2
  Mux2 : Mux  Inputs=2
  atan2((21/22)/cos) : Fcn  Expr=atan2(u[1],u[2])
  atan2(32/21) : Fcn  Expr=atan2(u[8],-u[4])
  Euler Angles : Outport  VectorParamsAs1DForOutWhenUnconnected=off
  wires:
  DCM/1 -> 22/1, 21/1, atan2(32/21)/1
  Mux/1 -> Euler Angles/1
  Constant/1 -> Mux/2
  atan2(32/21)/1 -> Mux/1, Mux1/1
  atan2((21/22)/cos)/1 -> Mux/3
  Mux1/1 -> (22*cos)/1
  22/1 -> Mux1/2
  Mux2/1 -> atan2((21/22)/cos)/1
  (22*cos)/1 -> Mux2/2
  21/1 -> Mux2/1

== system Latest_Greatest/Subsystem3/Subsystem1/312 ==
  note: y
  note: q
  note: f
  DCM : Inport
  (23*cos) : Fcn  Expr=u[2]*cos(u[1])
  23 : Fcn  Expr=u[6]
  33 : Fcn  Expr=u[9]
  Mux : Mux  Inputs=3
  Mux1 : Mux  Inputs=2
  Mux2 : Mux  Inputs=2
  atan2(13/33) : Fcn  Expr=atan2(-u[3],u[9])
  atan2(21/22) : Fcn  Expr=atan2(-u[4],u[5])
  atan2(23/33*cos) : Fcn  Expr=atan2(u[1],u[2])
  Euler Angles : Outport  VectorParamsAs1DForOutWhenUnconnected=off
  wires:
  atan2(21/22)/1 -> Mux/3
  DCM/1 -> atan2(21/22)/1, 23/1, atan2(13/33)/1, 33/1
  Mux/1 -> Euler Angles/1
  atan2(13/33)/1 -> Mux1/1, Mux/1
  atan2(23/33*cos)/1 -> Mux/2
  23/1 -> Mux1/2
  Mux1/1 -> (23*cos)/1
  Mux2/1 -> atan2(23/33*cos)/1
  33/1 -> Mux2/2
  (23*cos)/1 -> Mux2/1

== system Latest_Greatest/Subsystem3/Subsystem1/313 ==
  note: y
  note: q
  note: f
  DCM : Inport
  (33*sin) : Fcn  Expr=u[1]*sin(u[2])
  13 : Fcn  Expr=u[3]
  33 : Fcn  Expr=u[9]
  Constant : Constant  Value=0
  Mux : Mux  Inputs=3
  Mux1 : Mux  Inputs=2
  Mux2 : Mux  Inputs=2
  atan2((13/33)/sin) : Fcn  Expr=atan2(u[1],u[2])
  atan2(13/23) : Fcn  Expr=atan2(u[3],u[6])
  Euler Angles : Outport  VectorParamsAs1DForOutWhenUnconnected=off
  wires:
  DCM/1 -> 33/1, atan2(13/23)/1, 13/1
  Mux/1 -> Euler Angles/1
  Constant/1 -> Mux/1
  atan2(13/23)/1 -> Mux2/2, Mux/3
  atan2((13/33)/sin)/1 -> Mux/2
  Mux1/1 -> atan2((13/33)/sin)/1
  13/1 -> Mux1/1
  (33*sin)/1 -> Mux1/2
  33/1 -> Mux2/1
  Mux2/1 -> (33*sin)/1

== system Latest_Greatest/Subsystem3/Subsystem1/321 ==
  note: y
  note: f
  note: q
  note: f
  DCM : Inport
  31 : Fcn  Expr=u[7]
  31*cos(fi) : Fcn  Expr=u[1]*cos(u[2])
  33 : Fcn  Expr=u[9]
  Mux : Mux  Inputs=3
  Mux1 : Mux  Inputs=2
  Mux2 : Mux  Inputs=2
  atan2(21/11) : Fcn  Expr=atan2(-u[4],u[1])
  atan2(31/33*cos) : Fcn  Expr=atan2(u[1],u[2])
  atan2(32/33) : Fcn  Expr=atan2(-u[8],u[9])
  Euler Angles : Outport  VectorParamsAs1DForOutWhenUnconnected=off
  wires:
  atan2(21/11)/1 -> Mux/3
  atan2(32/33)/1 -> Mux/2, Mux1/2
  atan2(31/33*cos)/1 -> Mux/1
  DCM/1 -> atan2(21/11)/1, 33/1, 31/1, atan2(32/33)/1
  Mux/1 -> Euler Angles/1
  Mux1/1 -> 31*cos(fi)/1
  31/1 -> Mux1/1
  Mux2/1 -> atan2(31/33*cos)/1
  31*cos(fi)/1 -> Mux2/1
  33/1 -> Mux2/2

== system Latest_Greatest/Subsystem3/Subsystem1/323 ==
  note: y
  note: q
  note: f
  DCM : Inport
  (33*sin) : Fcn  Expr=u[1]*sin(u[2])
  32 : Fcn  Expr=u[8]
  33 : Fcn  Expr=u[9]
  Constant : Constant  Value=0
  Mux : Mux  Inputs=3
  Mux1 : Mux  Inputs=2
  Mux2 : Mux  Inputs=2
  atan2((32/33)/sin) : Fcn  Expr=atan2(u[1],u[2])
  atan2(32/31) : Fcn  Expr=atan2(u[8],u[7])
  Euler Angles : Outport  VectorParamsAs1DForOutWhenUnconnected=off
  wires:
  atan2(32/31)/1 -> Mux2/2, Mux/3
  DCM/1 -> atan2(32/31)/1, 33/1, 32/1
  Mux/1 -> Euler Angles/1
  Constant/1 -> Mux/2
  atan2((32/33)/sin)/1 -> Mux/1
  Mux2/1 -> (33*sin)/1
  33/1 -> Mux2/1
  (33*sin)/1 -> Mux1/2
  Mux1/1 -> atan2((32/33)/sin)/1
  32/1 -> Mux1/1

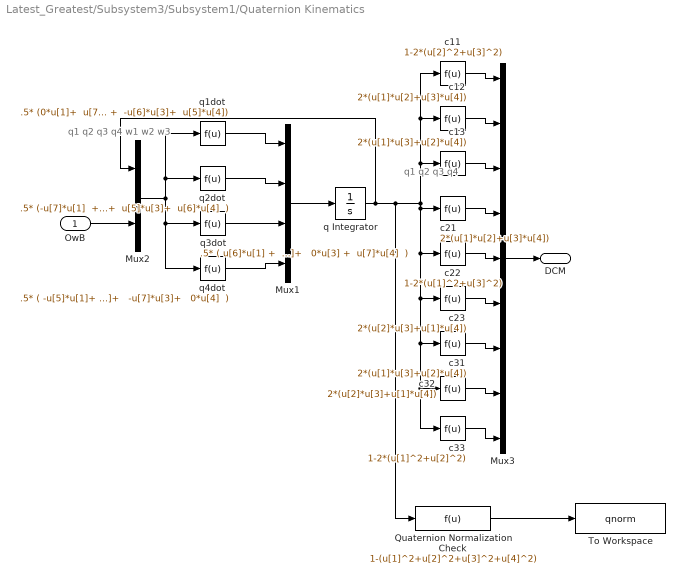
== system Latest_Greatest/Subsystem3/Subsystem1/Quaternion Kinematics ==
  note: q1
      | q2
      | q3
      | q4
      | w1
      | w2
      | w3
  note: q1
      | q2
      | q3
      | q4
  OwB : Inport
  Mux1 : Mux
  Mux2 : Mux  Inputs=2
  Mux3 : Mux  Inputs=9
  Quaternion Normalization Check : Fcn  Expr=1-(u[1]^2+u[2]^2+u[3]^2+u[4]^2)
  To Workspace : ToWorkspace  VariableName=qnorm  SaveFormat=Timeseries  SampleTime=-1
  c11 : Fcn  Expr=1-2*(u[2]^2+u[3]^2)
  c12 : Fcn  Expr=2*(u[1]*u[2]+u[3]*u[4])
  c13 : Fcn  Expr=2*(u[1]*u[3]+u[2]*u[4])
  c21 : Fcn  Expr=2*(u[1]*u[2]+u[3]*u[4])
  c22 : Fcn  Expr=1-2*(u[1]^2+u[3]^2)
  c23 : Fcn  Expr=2*(u[2]*u[3]+u[1]*u[4])
  c31 : Fcn  Expr=2*(u[1]*u[3]+u[2]*u[4])
  c32 : Fcn  Expr=2*(u[2]*u[3]+u[1]*u[4])
  c33 : Fcn  Expr=1-2*(u[1]^2+u[2]^2)
  q Integrator : Integrator  InitialCondition=qo
  q1dot : Fcn  Expr=".5* (0*u[1]+  u[7]*u[2] +  -u[6]*u[3]+  u[5]*u[4])"
  q2dot : Fcn  Expr=".5* (-u[7]*u[1]  +  0*u[2]+  u[5]*u[3]+  u[6]*u[4]  )"
  q3dot : Fcn  Expr=".5* ( u[6]*u[1] +  -u[5]*u[2]+   0*u[3] +  u[7]*u[4]  )"
  q4dot : Fcn  Expr=".5* ( -u[5]*u[1]+   -u[6]*u[2]+   -u[7]*u[3]+   0*u[4]  )"
  DCM : Outport  VectorParamsAs1DForOutWhenUnconnected=off
  wires:
  OwB/1 -> Mux2/2
  q1dot/1 -> Mux1/1
  q2dot/1 -> Mux1/2
  q3dot/1 -> Mux1/3
  q4dot/1 -> Mux1/4
  Mux1/1 -> q Integrator/1
  q Integrator/1 -> Quaternion Normalization Check/1, c12/1, c11/1, c13/1, c21/1, c22/1, c23/1, c31/1, c33/1, c32/1, Mux2/1
  c11/1 -> Mux3/1
  c12/1 -> Mux3/2
  c13/1 -> Mux3/3
  c22/1 -> Mux3/5
  c21/1 -> Mux3/4
  c23/1 -> Mux3/6
  c31/1 -> Mux3/7
  c32/1 -> Mux3/8
  c33/1 -> Mux3/9
  Mux3/1 -> DCM/1
  Mux2/1 -> q2dot/1, q1dot/1, q3dot/1, q4dot/1
  Quaternion Normalization Check/1 -> To Workspace/1

== system Latest_Greatest/Subsystem3/Subsystem1/Select ci2 ==
  U : Inport
  C12 : Fcn  Expr=u[2]
  C22 : Fcn  Expr=u[5]
  C32 : Fcn  Expr=u[8]
  Mux2 : Mux  Inputs=3
  U(E) : Outport  VectorParamsAs1DForOutWhenUnconnected=off
  wires:
  C12/1 -> Mux2/1
  C22/1 -> Mux2/2
  C32/1 -> Mux2/3
  U/1 -> C32/1, C22/1, C12/1
  Mux2/1 -> U(E)/1

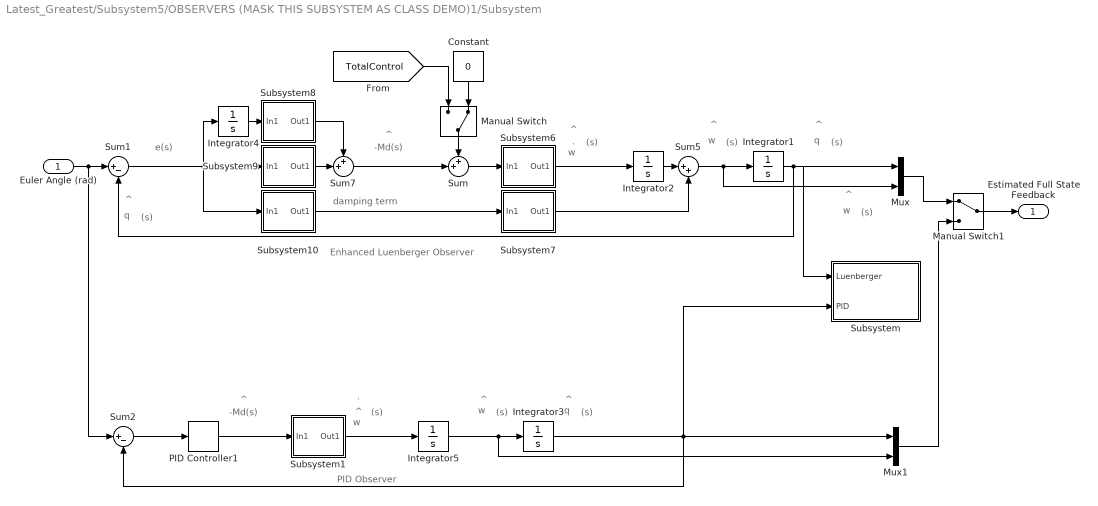
== system Latest_Greatest/Subsystem5/OBSERVERS (MASK THIS SUBSYSTEM AS CLASS DEMO)1/Subsystem ==
  note: PID Observer
  note: -Md(s)
  note: ^
  note: ^
  note: (s)
  note: w
  note: (s)
  note: .
  note: ^
  note: w
  note: e(s)
  note: q
  note: ^
  note: (s)
  note: ^
  note: (s)
  note: w
  note: damping term
  note: Enhanced Luenberger Observer
  note: ^
  note: (s)
  note: w
  note: (s)
  note: .
  note: ^
  note: w
  note: (s)
  note: ^
  note: q
  note: ^
  note: -Md(s)
  note: (s)
  note: ^
  note: q
  Euler Angle (rad) : Inport
  Constant : Constant  Value=0
  Integrator{1..5} (5 alike) : Integrator
  Manual Switch : ManualSwitch  CurrentSetting=0
  Manual Switch1 : ManualSwitch
  Mux : Mux  Inputs=2
  Mux1 : Mux  Inputs=2
  PID Controller1 : simulink_need_slupdate/PID Controller  P=Kpo  I=Kio  D=Kdo
  Subsystem : Subsystem
      mask Display: disp('Scopes')
  Subsystem1 : Subsystem
      mask Display: disp('1/J^p')
  Subsystem10 : Subsystem
      mask Display: disp('Kdo')
  Subsystem6 : Subsystem
      mask Display: disp('1/J^p')
  Subsystem7 : Subsystem
      mask Display: disp('1/J^p')
  Subsystem8 : Subsystem
      mask Display: disp('Kio')
  Subsystem9 : Subsystem
      mask Display: disp('Kpo')
  Sum : Sum  Inputs=++|
  Sum1 : Sum  Inputs=|+-
  Sum2 : Sum  Inputs=|+-
  Sum5 : Sum  Inputs=|++
  Sum7 : Sum  Inputs=++|
  Estimated Full State Feedback : Outport  VectorParamsAs1DForOutWhenUnconnected=off
  wires:
  Manual Switch1/1 -> Estimated Full State Feedback/1
  Mux1/1 -> Manual Switch1/2
  Mux/1 -> Manual Switch1/1
  PID Controller1/1 -> Subsystem1/1(In1)
  Integrator3/1 -> Mux1/1, Subsystem/2(PID), Sum2/2
  Integrator5/1 -> Mux1/2, Integrator3/1
  Subsystem1/1(Out1) -> Integrator5/1
  Manual Switch/1 -> Sum/1
  Constant/1 -> Manual Switch/2
  [TotalControl] -> Manual Switch/1
  Euler Angle (rad)/1 -> Sum1/1, Sum2/1
  Sum1/1 -> Subsystem10/1(In1), Subsystem9/1(In1), Integrator4/1
  Sum/1 -> Subsystem6/1(In1)
  Sum7/1 -> Sum/2
  Integrator1/1 -> Subsystem/1(Luenberger), Sum1/2, Mux/1
  Sum5/1 -> Mux/2, Integrator1/1
  Integrator4/1 -> Subsystem8/1(In1)
  Subsystem10/1(Out1) -> Subsystem7/1(In1)
  Subsystem9/1(Out1) -> Sum7/2
  Subsystem8/1(Out1) -> Sum7/1
  Subsystem7/1(Out1) -> Sum5/2
  Integrator2/1 -> Sum5/1
  Subsystem6/1(Out1) -> Integrator2/1
  Sum2/1 -> PID Controller1/1

== system Latest_Greatest/CMGs/Subsystem3/Subsystem1/Subsystem25 ==
  In1 : Inport
  Clock : Clock
  Ki : Gain  Gain=-Ki
  To Workspace : ToWorkspace  VariableName=t  SampleTime=-1
  Out1 : Outport  VectorParamsAs1DForOutWhenUnconnected=off
  wires:
  Clock/1 -> To Workspace/1
  In1/1 -> Ki/1
  Ki/1 -> Out1/1

== system Latest_Greatest/CMGs/Subsystem3/Subsystem1/Subsystem26 ==
  In1 : Inport
  Gain : Gain  Gain=-Kp
  Out1 : Outport  VectorParamsAs1DForOutWhenUnconnected=off
  wires:
  Gain/1 -> Out1/1
  In1/1 -> Gain/1

== system Latest_Greatest/CMGs/Subsystem3/Subsystem1/Subsystem27 ==
  In1 : Inport
  Gain : Gain  Gain=-Kd
  Out1 : Outport  VectorParamsAs1DForOutWhenUnconnected=off
  wires:
  In1/1 -> Gain/1
  Gain/1 -> Out1/1

== system Latest_Greatest/Subsystem2/Subsystem/Gravity Gradient/Select ci3 ==
  U : Inport
  C11 : Fcn  Expr=u[3]
  C12 : Fcn  Expr=u[6]
  C13 : Fcn  Expr=u[9]
  Mux2 : Mux  Inputs=3
  U(E) : Outport
  wires:
  Mux2/1 -> U(E)/1
  U/1 -> C13/1, C11/1, C12/1
  C13/1 -> Mux2/3
  C12/1 -> Mux2/2
  C11/1 -> Mux2/1

== system Latest_Greatest/Subsystem2/Subsystem/TAero & Tsolar/Select ci1 ==
  U : Inport
  C11 : Fcn  Expr=u[1]
  C21 : Fcn  Expr=u[4]
  C31 : Fcn  Expr=u[7]
  Mux2 : Mux  Inputs=3
  U(E) : Outport
  wires:
  Mux2/1 -> U(E)/1
  U/1 -> C31/1, C11/1, C21/1
  C31/1 -> Mux2/3
  C21/1 -> Mux2/2
  C11/1 -> Mux2/1

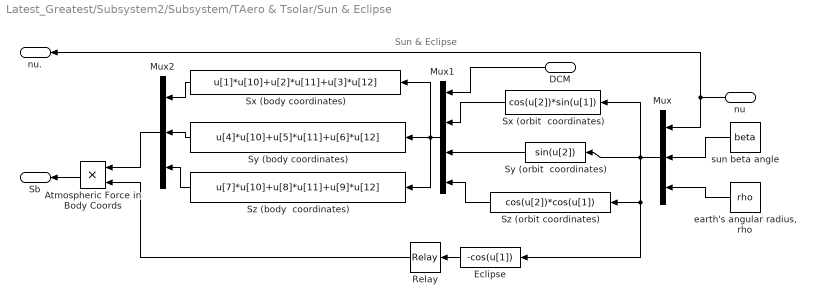
== system Latest_Greatest/Subsystem2/Subsystem/TAero & Tsolar/Sun & Eclipse ==
  note: Sun & Eclipse
  nu : Inport
  DCM : Inport  Port=2
  Atmospheric Force in Body Coords : Product  SaturateOnIntegerOverflow=on  OutDataTypeStr=Inherit: Same as first input
  Eclipse : Fcn  Expr=-cos(u[1])
  Mux : Mux  Inputs=3
  Mux1 : Mux
  Mux2 : Mux  Inputs=3
  Relay : Relay  OnSwitchValue=cos(rho)/cos(beta)  OffSwitchValue=cos(rho)/cos(beta)-0.001  OnOutputValue=0  OffOutputValue=1
  Sx (body coordinates) : Fcn  Expr=u[1]*u[10]+u[2]*u[11]+u[3]*u[12]
  Sx (orbit  coordinates) : Fcn  Expr=cos(u[2])*sin(u[1])
  Sy (body coordinates) : Fcn  Expr=u[4]*u[10]+u[5]*u[11]+u[6]*u[12]
  Sy (orbit  coordinates) : Fcn  Expr=sin(u[2])
  Sz (body  coordinates) : Fcn  Expr=u[7]*u[10]+u[8]*u[11]+u[9]*u[12]
  Sz (orbit coordinates) : Fcn  Expr=cos(u[2])*cos(u[1])
  "earth's angular radius, rho" : Constant  Value=rho
  sun beta angle : Constant  Value=beta
  Sb : Outport
  nu. : Outport  Port=2
  wires:
  DCM/1 -> Mux1/1
  Sz (orbit coordinates)/1 -> Mux1/4
  Sy (orbit  coordinates)/1 -> Mux1/3
  Sx (orbit  coordinates)/1 -> Mux1/2
  Mux2/1 -> Atmospheric Force in Body Coords/1
  Sz (body  coordinates)/1 -> Mux2/3
  Sy (body coordinates)/1 -> Mux2/2
  Sx (body coordinates)/1 -> Mux2/1
  Mux1/1 -> Sy (body coordinates)/1, Sz (body  coordinates)/1, Sx (body coordinates)/1
  Atmospheric Force in Body Coords/1 -> Sb/1
  nu/1 -> nu./1, Mux/1
  sun beta angle/1 -> Mux/2
  "earth's angular radius, rho"/1 -> Mux/3
  Mux/1 -> Sy (orbit  coordinates)/1, Sx (orbit  coordinates)/1, Sz (orbit coordinates)/1, Eclipse/1
  Eclipse/1 -> Relay/1
  Relay/1 -> Atmospheric Force in Body Coords/2

== system Latest_Greatest/Subsystem5/OBSERVERS (MASK THIS SUBSYSTEM AS CLASS DEMO)1/Subsystem/Subsystem ==
  Luenberger : Inport
  PID : Inport  Port=2
  Estimated Euler Angles (deg) : Scope
      settings: StopFcn=|
      | %Simulink figure properties
      | shh=get(0,'ShowHiddenHandles');
      | set(0,'ShowHiddenHandles','On')
      | set(gcf,'menubar','figure')
      | set(gcf,'CloseRequestFcn','closereq')
      | set(gcf,'DefaultLineClipping','Off')
      | set(0,'ShowHiddenHandles',shh)
  Reshape : Reshape
  Reshape2 : Reshape  OutputDimensions=[1,9]
  Reshape3 : Reshape  OutputDimensions=[1,9]
  Sum2 : Sum  Inputs=|+-
  Sum3 : Sum  Inputs=|+-
  To Workspace : ToWorkspace  VariableName=EstimatedEuler  SampleTime=-1
  To Workspace1 : ToWorkspace  VariableName=EstimationError  SampleTime=-1
  To Workspace2 : ToWorkspace  VariableName=PIDoEstimationError  SampleTime=-1
  degrees-to-radians1 : Gain  Gain=180/pi
  degrees-to-radians2 : Gain  Gain=180/pi
  wires:
  degrees-to-radians2/1 -> Reshape/1
  Reshape/1 -> Estimated Euler Angles (deg)/1, Sum3/2
  PID/1 -> degrees-to-radians2/1
  Sum3/1 -> To Workspace2/1
  Luenberger/1 -> degrees-to-radians1/1
  Reshape3/1 -> To Workspace1/1
  Reshape2/1 -> To Workspace/1
  [ActualEuler] -> Sum3/1, Sum2/1
  Sum2/1 -> Reshape3/1
  degrees-to-radians1/1 -> Reshape2/1, Sum2/2

== system Latest_Greatest/Subsystem5/OBSERVERS (MASK THIS SUBSYSTEM AS CLASS DEMO)1/Subsystem/Subsystem1 ==
  In1 : Inport
  Gain : Gain  Gain=Iinv  Multiplication=Matrix(K*u)
  Out1 : Outport  VectorParamsAs1DForOutWhenUnconnected=off
  wires:
  In1/1 -> Gain/1
  Gain/1 -> Out1/1

== system Latest_Greatest/Subsystem5/OBSERVERS (MASK THIS SUBSYSTEM AS CLASS DEMO)1/Subsystem/Subsystem10 ==
  In1 : Inport
  Gain : Gain  Gain=Kdo
  Out1 : Outport  VectorParamsAs1DForOutWhenUnconnected=off
  wires:
  Gain/1 -> Out1/1
  In1/1 -> Gain/1

== system Latest_Greatest/Subsystem5/OBSERVERS (MASK THIS SUBSYSTEM AS CLASS DEMO)1/Subsystem/Subsystem6 ==
  In1 : Inport
  Gain : Gain  Gain=Iinv  Multiplication=Matrix(K*u)
  Out1 : Outport  VectorParamsAs1DForOutWhenUnconnected=off
  wires:
  Gain/1 -> Out1/1
  In1/1 -> Gain/1

== system Latest_Greatest/Subsystem5/OBSERVERS (MASK THIS SUBSYSTEM AS CLASS DEMO)1/Subsystem/Subsystem7 ==
  In1 : Inport
  Gain : Gain  Gain=Iinv  Multiplication=Matrix(K*u)
  Out1 : Outport  VectorParamsAs1DForOutWhenUnconnected=off
  wires:
  In1/1 -> Gain/1
  Gain/1 -> Out1/1

== system Latest_Greatest/Subsystem5/OBSERVERS (MASK THIS SUBSYSTEM AS CLASS DEMO)1/Subsystem/Subsystem8 ==
  In1 : Inport
  Gain : Gain  Gain=Kio
  Out1 : Outport  VectorParamsAs1DForOutWhenUnconnected=off
  wires:
  Gain/1 -> Out1/1
  In1/1 -> Gain/1

== system Latest_Greatest/Subsystem5/OBSERVERS (MASK THIS SUBSYSTEM AS CLASS DEMO)1/Subsystem/Subsystem9 ==
  In1 : Inport
  Gain : Gain  Gain=Kpo
  Out1 : Outport  VectorParamsAs1DForOutWhenUnconnected=off
  wires:
  In1/1 -> Gain/1
  Gain/1 -> Out1/1
